simulink library "PES_CZ_FAW"  (Simulink 7.5)
settings: Solver=FixedStepDiscrete  StartTime=0.0  StopTime=10.0  FixedStep=0.01  MaxStep=0.01  RelTol=1e-3
undefined symbols (not defined in the file or in its folder): DiscIntNeverNeededParam, p_DRC_LoPsFilActPwr_s, p_DRC_LoPsFilPwrTi_s, p_DRC_LPFiltIC2_Tau_s, p_DRC_LPFiltIC2_Ts_s, p_DRC_LPFiltIC_Tau_s, p_DRC_LPFiltIC_Ts_s, Slope1, Slope2
libraries: BaseOperationLib_Browser x128, simulink x1
(part 1 of 2)
settings Model: Creator=ppr00086  LastModifiedBy=ppr00086

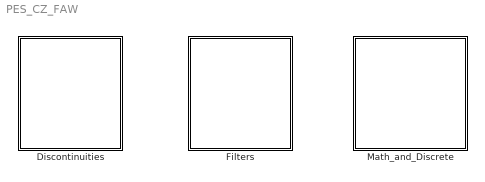
== system PES_CZ_FAW ==
  Discontinuities : Subsystem
  Filters : Subsystem  AncestorBlock=PES_CZ_FAW/Discontinuities
  Math_and_Discrete : Subsystem

== system PES_CZ_FAW/Discontinuities ==
  GetBit : Subsystem  mask{maska=16}
      mask prompts: maska "bitAND with parameter"
      mask help:
      | Get Bit
      |
      | Implements Masked AND between the input and mask. If the result is grater than zero true is set to output - otherwise false.
      |
      | Block is useful for decoding bit-encoded data.
      |
      | Mask may not be a calibratable parameter.
      mask Help:
      | Get Bit
      | 
      | Implements Masked AND between the input and mask. If the result is grater than zero true is set to output - otherwise false.
      | 
      | Block is useful for decoding bit-encoded data.
      | 
      | Mask may not be a calibratable parameter.
      mask Display: disp(['Input bitAND \n',maska]);
  Relay : Subsystem  mask{Thresshold=50, Hysteresis=5}
      mask help:
      | Block implements the relay functionality.
      |
      | Output is equal to one, when input is bigger or equal to Thresshold.
      | Output is equal to zero, when input is lower than (Thresshold - Hysteresis)
      | Otherwise, current output is equal to previous output.
      mask Help:
      | Block implements the relay functionality.
      | 
      | Output is equal to one, when input is bigger or equal to Thresshold.
      | Output is equal to zero, when input is lower than (Thresshold - Hysteresis)
      | Otherwise, current output is equal to previous output.
      mask Display: disp(['Relay']);
  SetBit : Subsystem  mask{maska=16}
      mask prompts: maska "Set to value"
      mask help:
      | Set Bit
      |
      | Sets the bit specified by value if the input is greater than zero.
      |
      | Block is useful for encoding bit-encoded data.
      |
      | "Set to value" may not be a calibratable parameter.
      mask Help:
      | Set Bit
      | 
      | Sets the bit specified by value if the input is greater than zero.
      | 
      | Block is useful for encoding bit-encoded data.
      | 
      | "Set to value" may not be a calibratable parameter.
      mask Display: disp(['SetBit \n',maska]);
  WrapToVal : Subsystem  mask{Max=1, Min=-1, Wrap=0}
      mask prompts: Wrap "WRAP TO VALUE"
      mask help: If the input is above the MAX or is less then MIN, the output is set to WRAP TO VALUE, otherwise the output equals the input.
      mask Display: disp('WrapTo', 'texmode', 'on');
  WtchDog : Subsystem  mask{timeoutthres=[]}
      mask prompts: timeoutthres "Timeout counter Treshold"
      mask help:
      | WatchDog block
      |
      | If input bool signal is false for the number of step bigger than "Timeout counter Threshold" the output WatchDog signal is set to True.
      |
      | Tip. Set the thresshold to the required time in seconds devided by algorithm sampling time.
      mask Help:
      | WatchDog block
      | 
      | If input bool signal is false for the number of step bigger than "Timeout counter Threshold" the output WatchDog signal is set to True.
      | 
      | Tip. Set the thresshold to required time in second devided by sampling time.
  valid_check : Subsystem  mask(Validity check      ){init=0}
      mask prompts: init "Init value"
      mask help:
      | Block checks, if the signal is valid. If not, signal is replaced by its
      | last valid value.
      mask Help:
      | Block checks, if the signal is valid. If not, signal is replaced by its
      | last valid value.

== system PES_CZ_FAW/Filters ==
  LPFilt : Subsystem  mask(Low-Pass filter){Ts=p_DRC_LoPsFilPwrTi_s, Tau=p_DRC_LoPsFilActPwr_s}
      mask prompts: Ts "Sampling Time Ts [s]"; Tau "Time constant Tau [s]"
      mask help:
      | Discrete low-pass filter of the first order that corresponds to continuous filter:
      |
      | T(s) = 1 / (Tau*s + 1)
      |
      | Filter is implemented using backward Euler discretization with sampling period Ts.
      |
      | For best results Tau and Ts should fullfill
      | Tau > 10 * Ts
      |
      | Note: Sampling rate of the filter inherrits the sampling rate of the input. This provides the compatibility with triggered subsystems.
      mask init:
      | if Ts*3>Tau,
      |    warndlg('Tau should be at least 3x higher than Ts')
      | end
      | 
      | if Tau<0,
      |    error('Tau must be greater than zero.')
      | end
      | 
      | if Ts<=0,
      |    error('Ts must be greater than zero.')
      | end
      settings: RTWSystemCode=Function  FunctionWithSeparateData=on
      mask Help:
      | Discrete low-pass filter of the first order that corresponds to continuous filter:
      | 
      | T(s) = 1 / (Tau*s + 1)
      | 
      | Filter is implemented using backward Euler discretization with sampling period Ts.
      | 
      | For best results Tau and Ts should fullfill
      | Tau > 10 * Ts
      | 
      | Note: Sampling rate of the filter inherrits the sampling rate of the input. This provides the compatibility with triggered subsystems.
      mask Display:
      | text(0.1,0.8,'1st order lowpass filter')
      | 
      | port_label('input',1,'u(t)')
      | 
      | port_label('output',1,'y(t)')
  LPFiltIC : Subsystem  mask(Low-Pass filter with external Initial Conditions){Ts=p_DRC_LPFiltIC_Ts_s, Tau=p_DRC_LPFiltIC_Tau_s}
      mask prompts: Ts "Sampling Time Ts [s]"; Tau "Time constant Tau [s]"
      mask help:
      | Discrete low-pass filter of the first order with external initial conditions that corresponds to continuous filter:
      |
      | T(s) = 1 / (Tau*s + 1)
      |
      | Filter is implemented using backward Euler discretization with sampling period Ts.
      |
      | For best results Tau and Ts should fullfill
      | Tau > 10 * Ts
      |
      | Note: Sampling rate of the filter inherrits the sampling rate of the input. This provides the compatibility with triggered subsystems.
      mask init:
      | if Ts*3>Tau,
      |    warndlg('Tau should be at least 3x higher than Ts')
      | end
      | 
      | if Tau<0,
      |    error('Tau must be greater than zero.')
      | end
      | 
      | if Ts<=0,
      |    error('Ts must be greater than zero.')
      | end
      settings: RTWSystemCode=Function  FunctionWithSeparateData=on
      mask Help:
      | Discrete low-pass filter of the first order that corresponds to continuous filter:
      | 
      | T(s) = 1 / (Tau*s + 1)
      | 
      | Filter is implemented using backward Euler discretization with sampling period Ts.
      | 
      | For best results Tau and Ts should fullfill
      | Tau > 10 * Ts
      | 
      | Note: Sampling rate of the filter inherrits the sampling rate of the input. This provides the compatibility with triggered subsystems.
      mask Display:
      | text(0.2,0.8,'1st order lowpass with IC');
      | 
      | port_label('input',1,'u(t)')
      | port_label('input',2,'IC')
      | port_label('output',1,'y(t)')
  LPFiltICEnRst : Subsystem  mask(Low-Pass filter Enabled Resettable External Initial Condition){Ts=p_DRC_LPFiltIC2_Ts_s, Tau=p_DRC_LPFiltIC2_Tau_s}
      mask prompts: Ts "Sampling Time Ts [s]"; Tau "Time constant Tau [s]"
      mask help:
      | Discrete low-pass filter of the first order with external initial conditions that corresponds to continuous filter:
      |
      | T(s) = 1 / (Tau*s + 1)
      |
      | Filter is implemented using backward Euler discretization with sampling period Ts.
      |
      | For best results Tau and Ts should fullfill
      | Tau > 10 * Ts
      |
      | The block is enabled, when the Enable input is equal to 1. The reset of the block is executed when the Reset input is set from 0 to 1.
      |
      | Note: Sampling rate of the filter inherrits the sampling rate of the input. This provides the compatibility with triggered subsystems.
      mask init:
      | if Ts*3>Tau,
      |    warndlg('Tau should be at least 3x higher than Ts')
      | end
      | 
      | if Tau<0,
      |    error('Tau must be greater than zero.')
      | end
      | 
      | if Ts<=0,
      |    error('Ts must be greater than zero.')
      | end
      mask Help:
      | Discrete low-pass filter of the first order that corresponds to continuous filter:
      | 
      | T(s) = 1 / (Tau*s + 1)
      | 
      | Filter is implemented using backward Euler discretization with sampling period Ts.
      | 
      | For best results Tau and Ts should fullfill
      | Tau > 10 * Ts
      | 
      | Note: Sampling rate of the filter inherrits the sampling rate of the input. This provides the compatibility with triggered subsystems.
      mask Display:
      | text(0.35,0.8,'1st order lowpass with IC');
      | text(0.35,0.25,strcat('Ts =',32,num2str(Ts),'s'));
      | text(0.35,0.5,strcat('Tau =',32,num2str(Tau),'s'));
      | 
      | port_label('input',1,'u(t)');
      | port_label('input',2,'IC')
      | port_label('output',1,'y(t)')
      | port_label('input',3,'Enable')
      | port_label('input',4,'Reset')
  LPFiltRst : Subsystem  mask(Low-Pass filter Resettable){Ts=[], Tau=[]}
      mask prompts: Ts "Sampling Time Ts [s]"; Tau "Time constant Tau [s]"
      mask help:
      | Discrete low-pass filter of the first order that corresponds to continuous filter:
      |
      | T(s) = 1 / (Tau*s + 1)
      |
      | Filter is implemented using backward Euler discretization with sampling period Ts.
      |
      | For best results Tau and Ts should fullfill
      | Tau > 10 * Ts
      |
      | Note: Sampling rate of the filter inherrits the sampling rate of the input. This provides the compatibility with triggered subsystems.
      mask init:
      | if Ts*3>Tau,
      |    warndlg('Tau should be at least 3x higher than Ts')
      | end
      | 
      | if Tau<0,
      |    error('Tau must be greater than zero.')
      | end
      | 
      | if Ts<=0,
      |    error('Ts must be greater than zero.')
      | end
      settings: RTWSystemCode=Function  FunctionWithSeparateData=on
      mask Help:
      | Discrete low-pass filter of the first order that corresponds to continuous filter:
      | 
      | T(s) = 1 / (Tau*s + 1)
      | 
      | Filter is implemented using backward Euler discretization with sampling period Ts.
      | 
      | For best results Tau and Ts should fullfill
      | Tau > 10 * Ts
      | 
      | Note: Sampling rate of the filter inherrits the sampling rate of the input. This provides the compatibility with triggered subsystems.
      mask Display:
      | text(0.25,0.8,'1st order lowpass');
      | text(0.25,0.25,strcat('Ts =',32,num2str(Ts),'s'));
      | text(0.25,0.5,strcat('Tau =',32,num2str(Tau),'s'));
  discrete_filter : Subsystem  mask(Discrete filter (first order)){num1=0, num2=0, den1=0, den2=0}
      mask prompts: num1 "num 1"; num2 "num 2"; den1 "den 1"; den2 "den 2"
      mask help:
      | num1*z + num2
      | Y(k) =  ------------------
      |            den1*z + den2
      mask Help:
      | num1*z + num2
      | Y(k) =  ------------------
      |            den1*z + den2
      mask Display:
      | port_label('input', 1, 'u(z)')
      | port_label('output', 1, 'y(z)')

== system PES_CZ_FAW/Math_and_Discrete ==
  Compare To Constant : Subsystem  mask(Compare To Constant){relop=<=, const=3.0, LogicOutDataTypeMode=uint8, ZeroCross=on}
      mask prompts: relop "Operator:"; const "Constant value:"; LogicOutDataTypeMode "Output data type mode:"; ZeroCross "Enable zero-crossing detection"
      mask help: Determine how a signal compares to a constant.
      mask init:
      | blkName = gcb;
      | 
      | if strcmp(get_param(gcbh,'LogicOutDataTypeMode'),'boolean')
      | 	setValue = 'Boolean';
      | else
      | 	setValue = 'Specify via dialog';
      | end
      | 
      | set_param([blkName,'/Compare'],'relop',relop, ...
      | 	'LogicOutDataTypeMode', setValue, 'ZeroCross', ZeroCross);
      | 
      | str = [relop,' C']; %default
      | 
      | const_str = get_param(blkName, 'const');
      | 
      | if isempty(strfind(const_str, ' ')) && isempty(strfind(const_str, ','))
      |     % scalar or single expression
      |     if isempty(str2num(const_str))
      |         %expression
      |         str = [relop, ' ', const_str];
      |     elseif length(const) == 1
      |         str = [relop,' ',num2str(double(const))];
      |     end
      | end
      mask StyleString: popup(==|~=|<|<=|>=|>),edit,popup(uint8|boolean),checkbox
      mask CallbackString: |||sl('zeroCrossEnable', gcbh);
      mask Display: disp(num2str(const));
  Compare To Zero : Subsystem  mask(Compare To Zero){relop=<=, LogicOutDataTypeMode=uint8, ZeroCross=on}
      mask prompts: relop "Operator:"; LogicOutDataTypeMode "Output data type mode:"; ZeroCross "Enable zero-crossing detection"
      mask help: Determine how a signal compares to zero.
      mask init:
      | blkName = gcb;
      | 
      | if strcmp(get_param(gcbh,'LogicOutDataTypeMode'),'boolean')
      | 	setValue = 'Boolean';
      | else
      |     setValue = 'Specify via dialog';
      | end
      | 
      | set_param([blkName,'/Compare'],'relop',relop, ...
      | 	'LogicOutDataTypeMode', setValue, 'ZeroCross', ZeroCross);
      mask StyleString: popup(==|~=|<|<=|>=|>),popup(uint8|boolean),checkbox
      mask CallbackString: ||sl('zeroCrossEnable', gcbh);
      mask Display: disp([relop,' 0'])
  Detect Decrease : Subsystem  mask(Detect Decrease){vinit=0.0}
      mask prompts: vinit "Initial condition:"
      mask help: If the input is strictly less than its previous value, then output TRUE, otherwise output FALSE. The initial condition determines the initial value of the previous input U/z.
      mask Display: fprintf('U < U/z')
  "Range Check " : Subsystem  mask(Range Checker){Min=0, Max=10}
      mask prompts: Min "Minumim"; Max "Maximum"
      mask help: Simple signal range check block. Checks whether the input signal falls into <Min,Max> interval.
      mask Help: Simple signal range check block. Checks whether the input signal falls into <Min,Max> interval.
  Rate Limiter Dynamic : Subsystem
      mask Type: Rate Limiter Dynamic
      mask Description: Limit rising and falling rates of the signals at the second input by using the first input (upper limit) and the third input (lower limit).
      mask Display: plot([0.15 0.95],[.5 .5],[.5 .5],[0.05 0.95],0.05+0.9*[.2 .8],0.05+0.9*[0 1]);
  Unit Delay Resettable : Subsystem  mask(Unit Delay Resettable){vinit=0, tsamp=-1}
      mask prompts: vinit "Initial Condition"; tsamp "Sample Time"
      mask help: Unit Delay Resettable
      mask Display: dpoly(1,[1 0],'z')

== system PES_CZ_FAW/Discontinuities/GetBit ==
  In1 : Inport  OutDataType=fixdt(1, 16)  OutScaling=2^0
  Bitwise Operator : S-Function  FunctionName=sfix_bitop  Parameters=UseBitMask,NumInputPorts,BitMask,BitMaskRealWorld,logicop  EnableBusSupport=off  mask(Bitwise Operator){logicop=AND, UseBitMask=on, NumInputPorts=1, BitMask=eval(maska), BitMaskRealWorld=Stored Integer}
      mask prompts: logicop "Operator:"; UseBitMask "Use bit mask ..."; NumInputPorts "Number of input ports:"; BitMask "Bit Mask"; BitMaskRealWorld "Treat mask as:"
      mask help: Perform the specified bitwise operation on the inputs. The output data type should represent zero exactly.
      mask init:
      | str = '';
      | if UseBitMask
      |   [m,n] = size(BitMask);
      |   if ischar(BitMask)
      |     len = m;
      |     n = 1;
      |   else
      |     len = m * n;
      |   end
      |   internalBitMask = zeros(m,n);
      |   if isnumeric(BitMask)
      |     for i=1:len,
      |       internalBitMask(i) = BitMask(i);
      |     end
      |   elseif ischar(BitMask)
      |     for i=1:m,
      |       internalBitMask(i) = hex2dec(BitMask(i,:));
      |     end
      |   elseif iscell(BitMask)
      |     for i=1:len,
      |       if isnumeric( BitMask{i} )
      |         internalBitMask(i) = BitMask{i};
      |       elseif ischar( BitMask{i} )
      |         internalBitMask(i) = hex2dec(BitMask{i});
      |       else
      |         errordlg(['Data type is not supported at cell item ', num2str(i) ]);
      |       end
      |     end
      |   end
      |   BitMask = internalBitMask;
      |   for i=1:len
      |     if BitMask(i) > (2^52)-1
      |       error(DAStudio.message('Simulink:blocks:BitMaskWordLengthTooLarge')); 
      |     end
      |   end 
      |   if len == 1
      |      if BitMaskRealWorld == 1 || BitMask(1) < 0
      |        str=num2str(BitMask(1));
      |      else
      |        str=['0x',dec2hex(floor(BitMask(1)))];
      |      end
      |   else
      |      str='Masks';
      |   end
      | else
      |   BitMask = 0;
      |   str='';
      | end
      mask StyleString: popup(AND|OR|NAND|NOR|XOR|NOT),checkbox,edit,edit,popup(Real World Value|Stored Integer)
      mask CallbackString: fixptdialog(gcbh)|fixptdialog(gcbh)|||
      mask Display: fprintf(['Bitwise\n',logicop,'\n',str])
  Compare To Constant : BaseOperationLib_Browser/Logic Operations Changed/Compare To Constant  SystemSampleTime=-1  relop=>  const=0
  Out1 : Outport  OutDataType=fixdt(1, 16)  OutScaling=2^0
  wires:
  In1/1 -> Bitwise Operator/1
  Bitwise Operator/1 -> Compare To Constant/1
  Compare To Constant/1 -> Out1/1

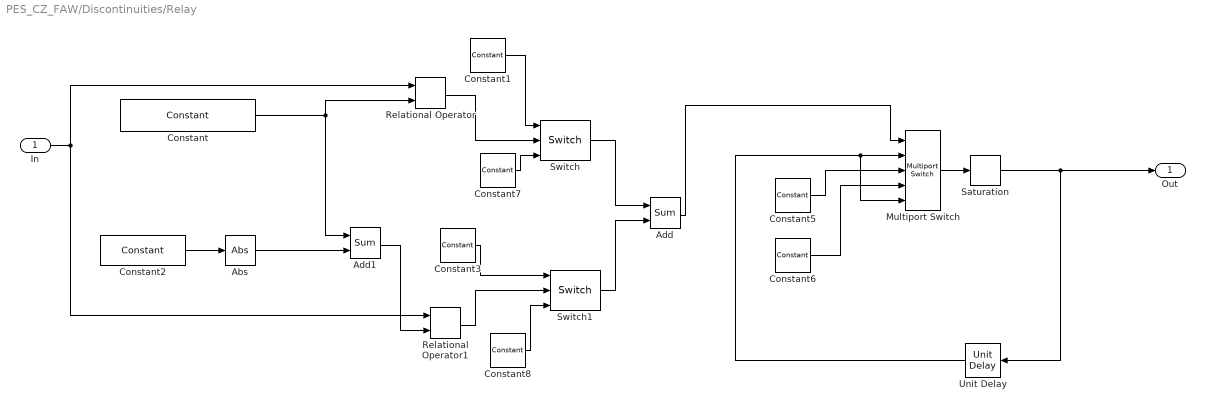
== system PES_CZ_FAW/Discontinuities/Relay ==
  In : Inport
  Abs : BaseOperationLib_Browser/Math Operations Changed/Abs  OutMax=[]  OutDataType=fixdt(1, 16)  OutScaling=2^0
  Add : BaseOperationLib_Browser/Math Operations Changed/Sum  Inputs=++  OutMin=[]  OutMax=[]  OutDataType=fixdt(1, 16)  OutScaling=2^0
  Add1 : BaseOperationLib_Browser/Math Operations Changed/Sum  Inputs=+-  OutMin=[]  OutMax=[]  OutDataType=fixdt(1, 16)  OutScaling=2^0
  Constant : BaseOperationLib_Browser/Sources&Sinks/Constant  Value=Thresshold  OutMin=[]  OutMax=[]  OutDataType=fixdt(1, 16)  ConRadixGroup=Use specified scaling  OutScaling=2^0  OutDataTypeStr=Inherit: Inherit from 'Constant value'
  Constant1 : BaseOperationLib_Browser/Sources&Sinks/Constant  Value=1  OutMin=[]  OutMax=[]  OutDataType=fixdt(1, 16)  ConRadixGroup=Use specified scaling  OutScaling=2^0  OutDataTypeStr=Inherit: Inherit from 'Constant value'
  Constant2 : BaseOperationLib_Browser/Sources&Sinks/Constant  Value=Hysteresis  OutMin=[]  OutMax=[]  OutDataType=fixdt(1, 16)  ConRadixGroup=Use specified scaling  OutScaling=2^0  OutDataTypeStr=Inherit: Inherit from 'Constant value'
  Constant3 : BaseOperationLib_Browser/Sources&Sinks/Constant  Value=2  OutMin=[]  OutMax=[]  OutDataType=fixdt(1, 16)  ConRadixGroup=Use specified scaling  OutScaling=2^0  OutDataTypeStr=Inherit: Inherit from 'Constant value'
  Constant5 : BaseOperationLib_Browser/Sources&Sinks/Constant  Value=1  OutMin=[]  OutMax=[]  OutDataType=fixdt(1, 16)  ConRadixGroup=Use specified scaling  OutScaling=2^0  OutDataTypeStr=Inherit: Inherit from 'Constant value'
  Constant6 : BaseOperationLib_Browser/Sources&Sinks/Constant  Value=0  OutMin=[]  OutMax=[]  OutDataType=fixdt(1, 16)  ConRadixGroup=Use specified scaling  OutScaling=2^0  OutDataTypeStr=Inherit: Inherit from 'Constant value'
  Constant7 : BaseOperationLib_Browser/Sources&Sinks/Constant  Value=0  OutMin=[]  OutMax=[]  OutDataType=fixdt(1, 16)  ConRadixGroup=Use specified scaling  OutScaling=2^0  OutDataTypeStr=Inherit: Inherit from 'Constant value'
  Constant8 : BaseOperationLib_Browser/Sources&Sinks/Constant  Value=0  OutMin=[]  OutMax=[]  OutDataType=fixdt(1, 16)  ConRadixGroup=Use specified scaling  OutScaling=2^0  OutDataTypeStr=Inherit: Inherit from 'Constant value'
  Multiport Switch : BaseOperationLib_Browser/Signal Routing Changed/Multiport Switch  DataPortOrder=Zero-based contiguous  Inputs=4  DataPortIndices={1,2,3}  zeroidx=on  OutMin=[]  OutMax=[]  OutDataType=fixdt(1, 16)  OutScaling=2^0
  Relational Operator : BaseOperationLib_Browser/Logic Operations Changed/Relational Operator  Operator=>=  LogicOutDataTypeMode=boolean  LogicDataType=PDT_Bool  OutDataTypeStr=boolean
  Relational Operator1 : BaseOperationLib_Browser/Logic Operations Changed/Relational Operator  Operator=<  LogicOutDataTypeMode=boolean  LogicDataType=PDT_Bool  OutDataTypeStr=boolean
  Saturation : BaseOperationLib_Browser/Discontinuities Unchanged/Saturation  UpperLimit=1  LowerLimit=0  OutMin=[]  OutMax=[]  OutDataType=fixdt(1, 16)  OutScaling=2^0
      settings: AttributesFormatString=ULim:%<UpperLimit>\nLLim:%<LowerLimit>
  Switch : BaseOperationLib_Browser/Signal Routing Changed/Switch  Criteria=u2 ~= 0  Threshold=0  OutMin=[]  OutMax=[]  OutDataType=fixdt(1,16,0)  OutScaling=[]
  Switch1 : BaseOperationLib_Browser/Signal Routing Changed/Switch  Criteria=u2 ~= 0  Threshold=0  OutMin=[]  OutMax=[]  OutDataType=fixdt(1,16,0)  OutScaling=[]
  Unit Delay : BaseOperationLib_Browser/Discrete Unchanged /Unit Delay  X0=0  SampleTime=-1
  Out : Outport
  wires:
  In/1 -> Relational Operator/1, Relational Operator1/1
  Constant/1 -> Add1/1, Relational Operator/2
  Relational Operator/1 -> Switch/2
  Constant1/1 -> Switch/1
  Relational Operator1/1 -> Switch1/2
  Constant3/1 -> Switch1/1
  Switch/1 -> Add/1
  Switch1/1 -> Add/2
  Add/1 -> Multiport Switch/1
  Abs/1 -> Add1/2
  Constant2/1 -> Abs/1
  Constant5/1 -> Multiport Switch/3
  Multiport Switch/1 -> Saturation/1
  Constant6/1 -> Multiport Switch/4
  Constant7/1 -> Switch/3
  Constant8/1 -> Switch1/3
  Unit Delay/1 -> Multiport Switch/2, Multiport Switch/5
  Saturation/1 -> Unit Delay/1, Out/1
  Add1/1 -> Relational Operator1/2

== system PES_CZ_FAW/Discontinuities/SetBit ==
  In1 : Inport  OutDataType=fixdt(1, 16)  OutScaling=2^0
  Compare To Constant : BaseOperationLib_Browser/Logic Operations Changed/Compare To Constant  SystemSampleTime=-1  relop=>  const=0
  Data Type Conversion : DataTypeConversion  OutDataTypeMode=uint32  OutDataType=fixdt(1, 16)  OutScaling=2^0  OutDataTypeStr=uint32
  Gain : BaseOperationLib_Browser/Math Operations Changed/Gain  Gain=uint32(eval(maska))  Multiplication=Element-wise(K.*u)  ParamMin=[]  ParamMax=[]  ParameterDataType=fixdt(1, 16)  ParameterScalingMode=Best Precision: Matrix-wise  ParameterScaling=2^0  ParamDataTypeStr=Inherit: Inherit from 'Gain'  OutMin=[]  OutMax=[]  OutDataType=fixdt(1, 16)  OutScaling=2^0  SaturateOnIntegerOverflow=on
  Out1 : Outport  OutDataType=fixdt(1, 16)  OutScaling=2^0
  wires:
  Compare To Constant/1 -> Data Type Conversion/1
  Gain/1 -> Out1/1
  In1/1 -> Compare To Constant/1
  Data Type Conversion/1 -> Gain/1

== system PES_CZ_FAW/Discontinuities/WrapToVal ==
  In1 : Inport  OutDataType=fixdt(1, 16)  OutScaling=2^0
  Compare To Constant : BaseOperationLib_Browser/Logic Operations Changed/Compare To Constant  SystemSampleTime=-1  relop=<=  const=Max
  Compare To Constant1 : BaseOperationLib_Browser/Logic Operations Changed/Compare To Constant  SystemSampleTime=-1  relop=>=  const=Min
  Constant : BaseOperationLib_Browser/Sources&Sinks/Constant  Value=Wrap  OutMin=[]  OutMax=[]  OutDataType=fixdt(1, 16)  ConRadixGroup=Use specified scaling  OutScaling=2^0  OutDataTypeStr=Inherit: Inherit via back propagation
  Logical Operator : BaseOperationLib_Browser/Logic Operations Changed/Logical Operator  Operator=AND  Inputs=2  AllPortsSameDT=on  OutDataTypeMode=Specify via dialog  LogicDataType=PDT_Bool  OutDataTypeStr=PDT_Bool
  Switch : BaseOperationLib_Browser/Signal Routing Changed/Switch  Criteria=u2 ~= 0  Threshold=1  InputSameDT=on  OutMin=[]  OutMax=[]  OutDataType=fixdt(1,16,0)  OutScaling=[]  SaturateOnIntegerOverflow=on
  Out1 : Outport  OutDataType=fixdt(1, 16)  OutScaling=2^0
  wires:
  In1/1 -> Compare To Constant1/1, Compare To Constant/1, Switch/1
  Switch/1 -> Out1/1
  Constant/1 -> Switch/3
  Logical Operator/1 -> Switch/2
  Compare To Constant1/1 -> Logical Operator/2
  Compare To Constant/1 -> Logical Operator/1

== system PES_CZ_FAW/Discontinuities/WtchDog ==
  ValidSig : Inport  OutDataType=fixdt(1, 16)  OutScaling=2^0
  Constant : BaseOperationLib_Browser/Sources&Sinks/Constant  Value=timeoutthres  OutMin=[]  OutMax=[]  OutDataType=fixdt(1, 16)  ConRadixGroup=Use specified scaling  OutScaling=2^0  OutDataTypeStr=Inherit: Inherit from 'Constant value'
  Discrete-Time Integrator1 : DiscreteIntegrator  IntegratorMethod=Integration: Backward Euler  ExternalReset=rising  SampleTime=-1  OutDataType=PDT_s  OutDataTypeStr=Inherit: Inherit via back propagation  UpperSaturationLimit=100  LowerSaturationLimit=0  ICPrevOutput=DiscIntNeverNeededParam  ICPrevScaledInput=DiscIntNeverNeededParam
  Logical Operator : BaseOperationLib_Browser/Logic Operations Changed/Logical Operator  Operator=AND  Inputs=2  AllPortsSameDT=on  OutDataTypeMode=Specify via dialog  LogicDataType=PDT_Bool  OutDataTypeStr=PDT_Bool
  Logical Operator2 : BaseOperationLib_Browser/Logic Operations Changed/Logical Operator  Operator=NOT  Inputs=2  AllPortsSameDT=on  OutDataTypeMode=Specify via dialog  LogicDataType=PDT_Bool  OutDataTypeStr=PDT_Bool
  Relational Operator : BaseOperationLib_Browser/Logic Operations Changed/Relational Operator  Operator=>=  InputSameDT=on  LogicOutDataTypeMode=Specify via dialog  LogicDataType=PDT_Bool  OutDataTypeStr=PDT_Bool
  WatchDogErr : Outport  OutDataType=fixdt(1, 16)  OutScaling=2^0
  wires:
  ValidSig/1 -> Logical Operator2/1
  Relational Operator/1 -> Logical Operator/1
  Logical Operator/1 -> WatchDogErr/1
  Constant/1 -> Relational Operator/2
  Discrete-Time Integrator1/1 -> Relational Operator/1
  Logical Operator2/1 -> Discrete-Time Integrator1/1, Discrete-Time Integrator1/2, Logical Operator/2

== system PES_CZ_FAW/Discontinuities/valid_check ==
  Signal : Inport
  Valid : Inport  Port=2
  Switch : BaseOperationLib_Browser/Signal Routing Changed/Switch  Criteria=u2 ~= 0  Threshold=1  InputSameDT=on  OutMin=[]  OutMax=[]  OutDataType=fixdt(1,16,0)  OutScaling=[]  SaturateOnIntegerOverflow=on
  Unit Delay : BaseOperationLib_Browser/Discrete Unchanged /Unit Delay  X0=init  SampleTime=-1
  SignalOut : Outport
  wires:
  Switch/1 -> Unit Delay/1, SignalOut/1
  Unit Delay/1 -> Switch/3
  Signal/1 -> Switch/1
  Valid/1 -> Switch/2

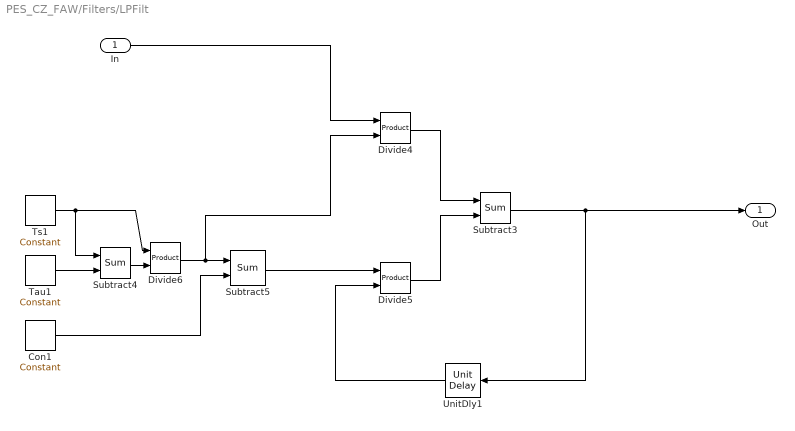
== system PES_CZ_FAW/Filters/LPFilt ==
  In : Inport
  Con1 : BaseOperationLib_Browser/Sources&Sinks/Constant  Value=1  OutMin=[]  OutMax=[]  OutDataType=fixdt(1, 16)  ConRadixGroup=Use specified scaling  OutScaling=2^0  OutDataTypeStr=Inherit: Inherit from 'Constant value'
  Divide4 : BaseOperationLib_Browser/Math Operations Changed/Product  Inputs=**  Multiplication=Element-wise(.*)  OutMin=[]  OutMax=[]  OutDataType=fixdt(1,16,0)  OutScaling=[]
  Divide5 : BaseOperationLib_Browser/Math Operations Changed/Product  Inputs=**  Multiplication=Element-wise(.*)  OutMin=[]  OutMax=[]  OutDataType=fixdt(1,16,0)  OutScaling=[]
  Divide6 : BaseOperationLib_Browser/Math Operations Changed/Product  Inputs=*/  Multiplication=Element-wise(.*)  OutMin=[]  OutMax=[]  OutDataType=fixdt(1,16,0)  OutScaling=[]
  Subtract3 : BaseOperationLib_Browser/Math Operations Changed/Sum  Inputs=++  OutMin=[]  OutMax=[]  OutDataType=fixdt(1, 16)  OutScaling=2^0
  Subtract4 : BaseOperationLib_Browser/Math Operations Changed/Sum  Inputs=++  OutMin=[]  OutMax=[]  OutDataType=fixdt(1, 16)  OutScaling=2^0
  Subtract5 : BaseOperationLib_Browser/Math Operations Changed/Sum  Inputs=-+  OutMin=[]  OutMax=[]  OutDataType=fixdt(1, 16)  OutScaling=2^0
  Tau1 : BaseOperationLib_Browser/Sources&Sinks/Constant  Value=Tau  OutMin=[]  OutMax=[]  OutDataType=fixdt(1, 16)  ConRadixGroup=Use specified scaling  OutScaling=2^0  OutDataTypeStr=Inherit: Inherit from 'Constant value'
  Ts1 : BaseOperationLib_Browser/Sources&Sinks/Constant  Value=Ts  OutMin=[]  OutMax=[]  OutDataType=fixdt(1, 16)  ConRadixGroup=Use specified scaling  OutScaling=2^0  OutDataTypeStr=Inherit: Inherit from 'Constant value'
  UnitDly1 : BaseOperationLib_Browser/Discrete Unchanged /Unit Delay  X0=0  SampleTime=-1
  Out : Outport
  wires:
  Subtract5/1 -> Divide5/1
  Tau1/1 -> Subtract4/2
  Ts1/1 -> Subtract4/1, Divide6/1
  Subtract4/1 -> Divide6/2
  Divide6/1 -> Divide4/2, Subtract5/1
  Con1/1 -> Subtract5/2
  In/1 -> Divide4/1
  Divide4/1 -> Subtract3/1
  UnitDly1/1 -> Divide5/2
  Divide5/1 -> Subtract3/2
  Subtract3/1 -> Out/1, UnitDly1/1

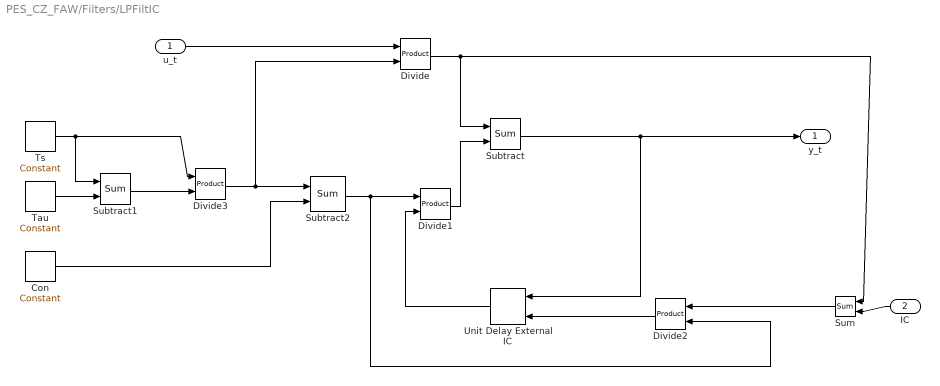
== system PES_CZ_FAW/Filters/LPFiltIC ==
  u_t : Inport
  IC : Inport  Port=2
  Con : BaseOperationLib_Browser/Sources&Sinks/Constant  Value=1  OutMin=[]  OutMax=[]  OutDataType=fixdt(1, 16)  ConRadixGroup=Use specified scaling  OutScaling=2^0  OutDataTypeStr=Inherit: Inherit from 'Constant value'
  Divide : BaseOperationLib_Browser/Math Operations Changed/Product  Inputs=**  Multiplication=Element-wise(.*)  OutMin=[]  OutMax=[]  OutDataType=fixdt(1,16,0)  OutScaling=[]
  Divide1 : BaseOperationLib_Browser/Math Operations Changed/Product  Inputs=**  Multiplication=Element-wise(.*)  OutMin=[]  OutMax=[]  OutDataType=fixdt(1,16,0)  OutScaling=[]
  Divide2 : BaseOperationLib_Browser/Math Operations Changed/Product  Inputs=*/  Multiplication=Element-wise(.*)  OutMin=[]  OutMax=[]  OutDataType=fixdt(1,16,0)  OutScaling=[]
  Divide3 : BaseOperationLib_Browser/Math Operations Changed/Product  Inputs=*/  Multiplication=Element-wise(.*)  OutMin=[]  OutMax=[]  OutDataType=fixdt(1,16,0)  OutScaling=[]
  Subtract : BaseOperationLib_Browser/Math Operations Changed/Sum  Inputs=++  OutMin=[]  OutMax=[]  OutDataType=fixdt(1, 16)  OutScaling=2^0
  Subtract1 : BaseOperationLib_Browser/Math Operations Changed/Sum  Inputs=++  OutMin=[]  OutMax=[]  OutDataType=fixdt(1, 16)  OutScaling=2^0
  Subtract2 : BaseOperationLib_Browser/Math Operations Changed/Sum  Inputs=-+  OutMin=[]  OutMax=[]  OutDataType=fixdt(1, 16)  OutScaling=2^0
  Sum : BaseOperationLib_Browser/Math Operations Changed/Sum  Inputs=-+|  OutMin=[]  OutMax=[]  OutDataType=fixdt(1, 16)  OutScaling=2^0
  Tau : BaseOperationLib_Browser/Sources&Sinks/Constant  Value=Tau  OutMin=[]  OutMax=[]  OutDataType=fixdt(1, 16)  ConRadixGroup=Use specified scaling  OutScaling=2^0  OutDataTypeStr=Inherit: Inherit from 'Constant value'
  Ts : BaseOperationLib_Browser/Sources&Sinks/Constant  Value=Ts  OutMin=[]  OutMax=[]  OutDataType=fixdt(1, 16)  ConRadixGroup=Use specified scaling  OutScaling=2^0  OutDataTypeStr=Inherit: Inherit from 'Constant value'
  Unit Delay External IC : BaseOperationLib_Browser/Discrete Unchanged /Unit Delay External IC  SystemSampleTime=-1  tsamp=-1
  y_t : Outport
  wires:
  Tau/1 -> Subtract1/2
  Ts/1 -> Subtract1/1, Divide3/1
  Subtract1/1 -> Divide3/2
  Divide3/1 -> Divide/2, Subtract2/1
  Con/1 -> Subtract2/2
  Subtract2/1 -> Divide2/2, Divide1/1
  IC/1 -> Sum/2
  Sum/1 -> Divide2/1
  Divide2/1 -> Unit Delay External IC/2
  u_t/1 -> Divide/1
  Divide/1 -> Sum/1, Subtract/1
  Unit Delay External IC/1 -> Divide1/2
  Divide1/1 -> Subtract/2
  Subtract/1 -> Unit Delay External IC/1, y_t/1

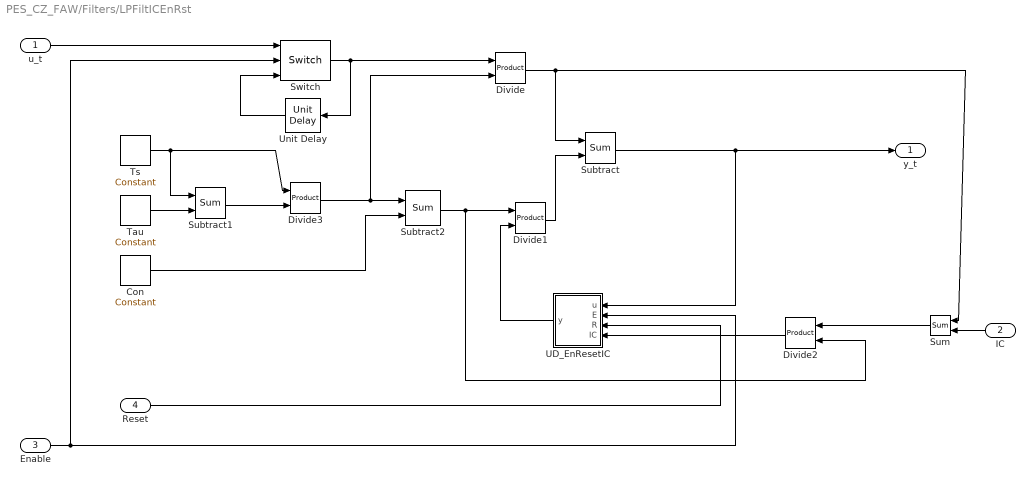
== system PES_CZ_FAW/Filters/LPFiltICEnRst ==
  u_t : Inport
  IC : Inport  Port=2
  Enable : Inport  Port=3
  Reset : Inport  Port=4
  Con : BaseOperationLib_Browser/Sources&Sinks/Constant  Value=1  OutMin=[]  OutMax=[]  OutDataType=fixdt(1, 16)  ConRadixGroup=Use specified scaling  OutScaling=2^0  OutDataTypeStr=Inherit: Inherit from 'Constant value'
  Divide : BaseOperationLib_Browser/Math Operations Changed/Product  Inputs=**  Multiplication=Element-wise(.*)  OutMin=[]  OutMax=[]  OutDataType=fixdt(1,16,0)  OutScaling=[]
  Divide1 : BaseOperationLib_Browser/Math Operations Changed/Product  Inputs=**  Multiplication=Element-wise(.*)  OutMin=[]  OutMax=[]  OutDataType=fixdt(1,16,0)  OutScaling=[]
  Divide2 : BaseOperationLib_Browser/Math Operations Changed/Product  Inputs=*/  Multiplication=Element-wise(.*)  OutMin=[]  OutMax=[]  OutDataType=fixdt(1,16,0)  OutScaling=[]
  Divide3 : BaseOperationLib_Browser/Math Operations Changed/Product  Inputs=*/  Multiplication=Element-wise(.*)  OutMin=[]  OutMax=[]  OutDataType=fixdt(1,16,0)  OutScaling=[]
  Subtract : BaseOperationLib_Browser/Math Operations Changed/Sum  Inputs=++  OutMin=[]  OutMax=[]  OutDataType=fixdt(1, 16)  OutScaling=2^0
  Subtract1 : BaseOperationLib_Browser/Math Operations Changed/Sum  Inputs=++  OutMin=[]  OutMax=[]  OutDataType=fixdt(1, 16)  OutScaling=2^0
  Subtract2 : BaseOperationLib_Browser/Math Operations Changed/Sum  Inputs=-+  OutMin=[]  OutMax=[]  OutDataType=fixdt(1, 16)  OutScaling=2^0
  Sum : BaseOperationLib_Browser/Math Operations Changed/Sum  Inputs=-+  OutMin=[]  OutMax=[]  OutDataType=fixdt(1, 16)  OutScaling=2^0
  Switch : BaseOperationLib_Browser/Signal Routing Changed/Switch  Criteria=u2 > Threshold  Threshold=0  OutMin=[]  OutMax=[]  OutDataType=fixdt(1,16,0)  OutScaling=[]
  Tau : BaseOperationLib_Browser/Sources&Sinks/Constant  Value=Tau  OutMin=[]  OutMax=[]  OutDataType=fixdt(1, 16)  ConRadixGroup=Use specified scaling  OutScaling=2^0  OutDataTypeStr=Inherit: Inherit from 'Constant value'
  Ts : BaseOperationLib_Browser/Sources&Sinks/Constant  Value=Ts  OutMin=[]  OutMax=[]  OutDataType=fixdt(1, 16)  ConRadixGroup=Use specified scaling  OutScaling=2^0  OutDataTypeStr=Inherit: Inherit from 'Constant value'
  UD_EnResetIC : Subsystem
  Unit Delay : BaseOperationLib_Browser/Discrete Unchanged /Unit Delay  X0=0  SampleTime=-1
  y_t : Outport
  wires:
  Con/1 -> Subtract2/2
  Divide3/1 -> Subtract2/1, Divide/2
  Subtract1/1 -> Divide3/2
  Ts/1 -> Divide3/1, Subtract1/1
  Tau/1 -> Subtract1/2
  Reset/1 -> UD_EnResetIC/3(R)
  Enable/1 -> Switch/2, UD_EnResetIC/2(E)
  Divide2/1 -> UD_EnResetIC/4(IC)
  Subtract/1 -> UD_EnResetIC/1(u), y_t/1
  Divide1/1 -> Subtract/2
  UD_EnResetIC/1(y) -> Divide1/2
  Divide/1 -> Subtract/1, Sum/1
  Sum/1 -> Divide2/1
  IC/1 -> Sum/2
  Subtract2/1 -> Divide1/1, Divide2/2
  Unit Delay/1 -> Switch/3
  u_t/1 -> Switch/1
  Switch/1 -> Divide/1, Unit Delay/1

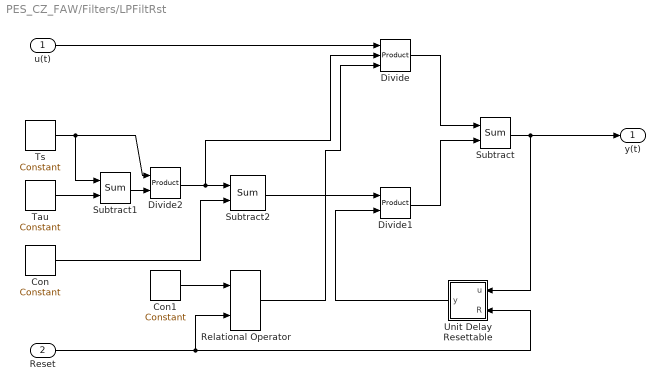
== system PES_CZ_FAW/Filters/LPFiltRst ==
  u(t) : Inport
  Reset : Inport  Port=2
  Con : BaseOperationLib_Browser/Sources&Sinks/Constant  Value=1  OutMin=[]  OutMax=[]  OutDataType=fixdt(1, 16)  ConRadixGroup=Use specified scaling  OutScaling=2^0  OutDataTypeStr=Inherit: Inherit from 'Constant value'
  Con1 : BaseOperationLib_Browser/Sources&Sinks/Constant  Value=0  OutMin=[]  OutMax=[]  OutDataType=fixdt(1, 16)  ConRadixGroup=Use specified scaling  OutScaling=2^0  OutDataTypeStr=Inherit: Inherit via back propagation
  Divide : BaseOperationLib_Browser/Math Operations Changed/Product  Inputs=***  Multiplication=Element-wise(.*)  OutMin=[]  OutMax=[]  OutDataType=fixdt(1,16,0)  OutScaling=[]
  Divide1 : BaseOperationLib_Browser/Math Operations Changed/Product  Inputs=**  Multiplication=Element-wise(.*)  OutMin=[]  OutMax=[]  OutDataType=fixdt(1,16,0)  OutScaling=[]
  Divide2 : BaseOperationLib_Browser/Math Operations Changed/Product  Inputs=*/  Multiplication=Element-wise(.*)  OutMin=[]  OutMax=[]  OutDataType=fixdt(1,16,0)  OutScaling=[]
  Relational Operator : BaseOperationLib_Browser/Logic Operations Changed/Relational Operator  Operator===  InputSameDT=on  LogicOutDataTypeMode=Specify via dialog  LogicDataType=PDT_Bool  OutDataTypeStr=PDT_Bool
  Subtract : BaseOperationLib_Browser/Math Operations Changed/Sum  Inputs=++  OutMin=[]  OutMax=[]  OutDataType=fixdt(1, 16)  OutScaling=2^0
  Subtract1 : BaseOperationLib_Browser/Math Operations Changed/Sum  Inputs=++  OutMin=[]  OutMax=[]  OutDataType=fixdt(1, 16)  OutScaling=2^0
  Subtract2 : BaseOperationLib_Browser/Math Operations Changed/Sum  Inputs=-+  OutMin=[]  OutMax=[]  OutDataType=fixdt(1, 16)  OutScaling=2^0
  Tau : BaseOperationLib_Browser/Sources&Sinks/Constant  Value=Tau  OutMin=[]  OutMax=[]  OutDataType=fixdt(1, 16)  ConRadixGroup=Use specified scaling  OutScaling=2^0  OutDataTypeStr=Inherit: Inherit from 'Constant value'
  Ts : BaseOperationLib_Browser/Sources&Sinks/Constant  Value=Ts  OutMin=[]  OutMax=[]  OutDataType=fixdt(1, 16)  ConRadixGroup=Use specified scaling  OutScaling=2^0  OutDataTypeStr=Inherit: Inherit from 'Constant value'
  Unit Delay Resettable : Subsystem
  y(t) : Outport
  wires:
  Con1/1 -> Relational Operator/1
  Relational Operator/1 -> Divide/3
  Subtract2/1 -> Divide1/1
  Tau/1 -> Subtract1/2
  Ts/1 -> Subtract1/1, Divide2/1
  Subtract1/1 -> Divide2/2
  Divide2/1 -> Divide/2, Subtract2/1
  Con/1 -> Subtract2/2
  u(t)/1 -> Divide/1
  Divide/1 -> Subtract/1
  Unit Delay Resettable/1(y) -> Divide1/2
  Divide1/1 -> Subtract/2
  Subtract/1 -> y(t)/1, Unit Delay Resettable/1(u)
  Reset/1 -> Relational Operator/2, Unit Delay Resettable/2(R)

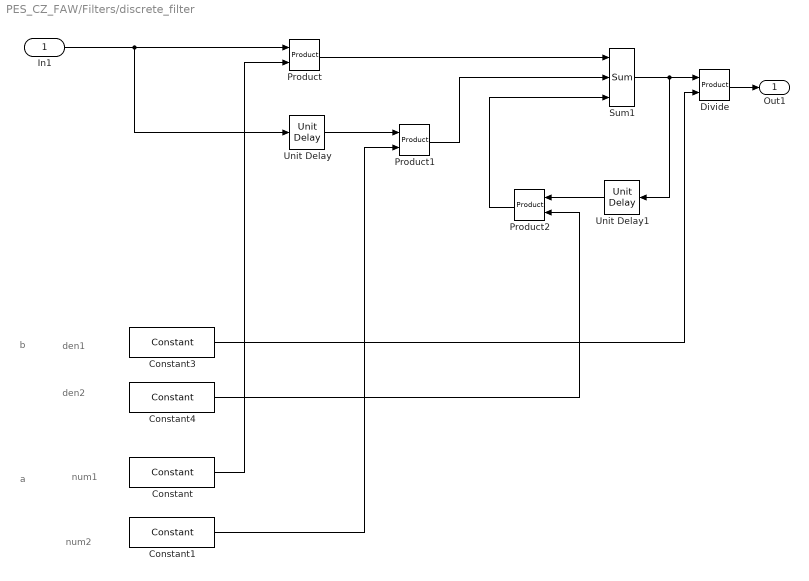
== system PES_CZ_FAW/Filters/discrete_filter ==
  note: b
  note: a
  note: den1
  note: den2
  note: num1
  note: num2
  In1 : Inport
  Constant : BaseOperationLib_Browser/Sources&Sinks/Constant  Value=num1  OutMin=[]  OutMax=[]  OutDataType=fixdt(1, 16)  ConRadixGroup=Use specified scaling  OutScaling=2^0  OutDataTypeStr=Inherit: Inherit from 'Constant value'
  Constant1 : BaseOperationLib_Browser/Sources&Sinks/Constant  Value=num2  OutMin=[]  OutMax=[]  OutDataType=fixdt(1, 16)  ConRadixGroup=Use specified scaling  OutScaling=2^0  OutDataTypeStr=Inherit: Inherit from 'Constant value'
  Constant3 : BaseOperationLib_Browser/Sources&Sinks/Constant  Value=den1  OutMin=[]  OutMax=[]  OutDataType=fixdt(1, 16)  ConRadixGroup=Use specified scaling  OutScaling=2^0  OutDataTypeStr=Inherit: Inherit from 'Constant value'
  Constant4 : BaseOperationLib_Browser/Sources&Sinks/Constant  Value=den2  OutMin=[]  OutMax=[]  OutDataType=fixdt(1, 16)  ConRadixGroup=Use specified scaling  OutScaling=2^0  OutDataTypeStr=Inherit: Inherit from 'Constant value'
  Divide : BaseOperationLib_Browser/Math Operations Changed/Product  Inputs=*/  Multiplication=Element-wise(.*)  OutMin=[]  OutMax=[]  OutDataType=fixdt(1,16,0)  OutScaling=[]
  Product : BaseOperationLib_Browser/Math Operations Changed/Product  Inputs=2  Multiplication=Element-wise(.*)  OutMin=[]  OutMax=[]  OutDataType=fixdt(1,16,0)  OutScaling=[]  OutDataTypeStr=Inherit: Inherit via back propagation  RndMeth=Zero  SaturateOnIntegerOverflow=on
  Product1 : BaseOperationLib_Browser/Math Operations Changed/Product  Inputs=2  Multiplication=Element-wise(.*)  OutMin=[]  OutMax=[]  OutDataType=fixdt(1,16,0)  OutScaling=[]  OutDataTypeStr=Inherit: Inherit via back propagation  RndMeth=Zero  SaturateOnIntegerOverflow=on
  Product2 : BaseOperationLib_Browser/Math Operations Changed/Product  Inputs=2  Multiplication=Element-wise(.*)  OutMin=[]  OutMax=[]  OutDataType=fixdt(1,16,0)  OutScaling=[]  OutDataTypeStr=Inherit: Inherit via back propagation  RndMeth=Zero  SaturateOnIntegerOverflow=on
  Sum1 : BaseOperationLib_Browser/Math Operations Changed/Sum  Inputs=++-  InputSameDT=on  OutMin=[]  OutMax=[]  OutDataType=fixdt(1, 16)  OutScaling=2^0  SaturateOnIntegerOverflow=on
  Unit Delay : BaseOperationLib_Browser/Discrete Unchanged /Unit Delay  X0=0  SampleTime=-1
  Unit Delay1 : BaseOperationLib_Browser/Discrete Unchanged /Unit Delay  X0=0  SampleTime=-1
  Out1 : Outport
  wires:
  Divide/1 -> Out1/1
  Constant3/1 -> Divide/2
  Product2/1 -> Sum1/3
  Constant4/1 -> Product2/2
  Unit Delay1/1 -> Product2/1
  Sum1/1 -> Divide/1, Unit Delay1/1
  Product1/1 -> Sum1/2
  Product/1 -> Sum1/1
  Constant1/1 -> Product1/2
  Unit Delay/1 -> Product1/1
  Constant/1 -> Product/2
  In1/1 -> Unit Delay/1, Product/1

== system PES_CZ_FAW/Math_and_Discrete/Compare To Constant ==
  u : Inport
  Constant : BaseOperationLib_Browser/Sources&Sinks/Constant  Value=const  OutMin=[]  OutMax=[]  OutDataType=fixdt(1, 16)  ConRadixGroup=Use specified scaling  OutScaling=2^0  OutDataTypeStr=Inherit: Inherit from 'Constant value'
  Relational Operator : BaseOperationLib_Browser/Logic Operations Changed/Relational Operator  Operator=<=  InputSameDT=on  LogicOutDataTypeMode=Specify via dialog  LogicDataType=PDT_Bool  OutDataTypeStr=PDT_Bool
  y : Outport
  wires:
  u/1 -> Relational Operator/1
  Constant/1 -> Relational Operator/2
  Relational Operator/1 -> y/1

== system PES_CZ_FAW/Math_and_Discrete/Compare To Zero ==
  u : Inport
  Constant : BaseOperationLib_Browser/Sources&Sinks/Constant  Value=0  OutMin=[]  OutMax=[]  OutDataType=fixdt(1, 16)  ConRadixGroup=Use specified scaling  OutScaling=2^0  OutDataTypeStr=Inherit: Inherit from 'Constant value'
  Relational Operator : BaseOperationLib_Browser/Logic Operations Changed/Relational Operator  Operator=<=  InputSameDT=on  LogicOutDataTypeMode=Specify via dialog  LogicDataType=PDT_Bool  OutDataTypeStr=PDT_Bool
  y : Outport
  wires:
  u/1 -> Relational Operator/1
  Constant/1 -> Relational Operator/2
  Relational Operator/1 -> y/1

== system PES_CZ_FAW/Math_and_Discrete/Detect Decrease ==
  U : Inport
  Relational Operator : RelationalOperator  Operator=<  LogicOutDataTypeMode=Specify via dialog  LogicDataType=PDT_Bool  OutDataTypeStr=PDT_Bool  InputSameDT=on
      mask Display: patch([0 1 1 1 .75], [1 1 0 .75 1], [0 1 0]);
  Unit Delay : UnitDelay  X0=vinit  SampleTime=-1
      mask Display: patch([0 1 1 1 .75], [1 1 0 .75 1], [0 1 0]);
  Y : Outport
  wires:
  U/1 -> Relational Operator/1, Unit Delay/1
  Unit Delay/1 -> Relational Operator/2
  Relational Operator/1 -> Y/1

== system PES_CZ_FAW/Math_and_Discrete/Range Check  ==
  in : Inport
  Constant : BaseOperationLib_Browser/Sources&Sinks/Constant  Value=Max  OutMin=[]  OutMax=[]  OutDataType=fixdt(1, 16)  ConRadixGroup=Use specified scaling  OutScaling=2^0  OutDataTypeStr=Inherit: Inherit from 'Constant value'
  Constant1 : BaseOperationLib_Browser/Sources&Sinks/Constant  Value=Min  OutMin=[]  OutMax=[]  OutDataType=fixdt(1, 16)  ConRadixGroup=Use specified scaling  OutScaling=2^0  OutDataTypeStr=Inherit: Inherit from 'Constant value'
  Logical Operator : BaseOperationLib_Browser/Logic Operations Changed/Logical Operator  Operator=AND  Inputs=2  AllPortsSameDT=on  OutDataTypeMode=Specify via dialog  LogicDataType=PDT_Bool  OutDataTypeStr=PDT_Bool
  Relational Operator1 : BaseOperationLib_Browser/Logic Operations Changed/Relational Operator  Operator=>=  InputSameDT=on  LogicOutDataTypeMode=Specify via dialog  LogicDataType=PDT_Bool  OutDataTypeStr=PDT_Bool
  Relational Operator2 : BaseOperationLib_Browser/Logic Operations Changed/Relational Operator  Operator=<=  InputSameDT=on  LogicOutDataTypeMode=Specify via dialog  LogicDataType=PDT_Bool  OutDataTypeStr=PDT_Bool
  out : Outport
  wires:
  Logical Operator/1 -> out/1
  Constant/1 -> Relational Operator2/2
  in/1 -> Relational Operator1/1, Relational Operator2/1
  Constant1/1 -> Relational Operator1/2
  Relational Operator2/1 -> Logical Operator/2
  Relational Operator1/1 -> Logical Operator/1

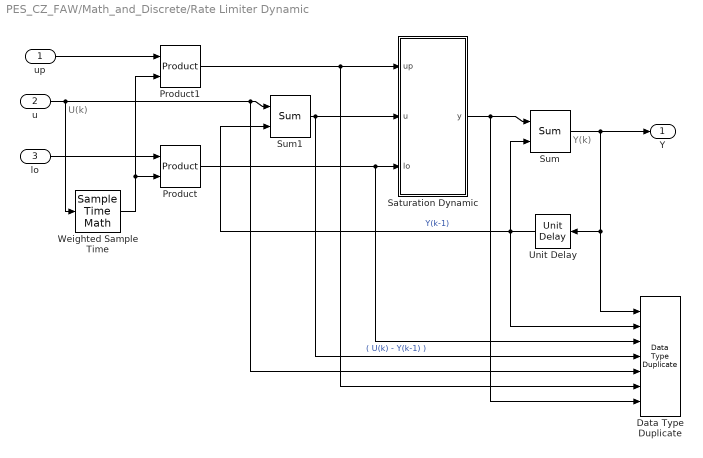
== system PES_CZ_FAW/Math_and_Discrete/Rate Limiter Dynamic ==
  note: Y(k)
  note: U(k)
  up : Inport  OutDataType=fixdt(1, 16)  OutScaling=2^0
  u : Inport  Port=2  OutDataType=fixdt(1, 16)  OutScaling=2^0
  lo : Inport  Port=3  OutDataType=fixdt(1, 16)  OutScaling=2^0
  Data Type Duplicate : DataTypeDuplicate  NumInputPorts=7
  Product : BaseOperationLib_Browser/Math Operations Changed/Product  Inputs=2  Multiplication=Element-wise(.*)  OutMin=[]  OutMax=[]  OutDataType=fixdt(1,16,0)  OutScaling=[]  OutDataTypeStr=Inherit: Inherit via back propagation  RndMeth=Zero  SaturateOnIntegerOverflow=on
  Product1 : BaseOperationLib_Browser/Math Operations Changed/Product  Inputs=2  Multiplication=Element-wise(.*)  OutMin=[]  OutMax=[]  OutDataType=fixdt(1,16,0)  OutScaling=[]  OutDataTypeStr=Inherit: Inherit via back propagation  RndMeth=Zero  SaturateOnIntegerOverflow=on
  Saturation Dynamic : Subsystem  mask(Saturation Dynamic){OutMin=[], OutMax=[], OutDataTypeStr=Inherit: Same as second input, OutputDataTypeScalingMode=Same as second input, OutDataType=fixdt(1, 16), OutScaling=2^-10, LockScale=off, RndMeth=Floor, DoSatur=off}
      mask prompts: OutMin "Output minimum:"; OutMax "Output maximum:"; OutDataTypeStr "Output data type:"; OutputDataTypeScalingMode "Output data type mode:"; OutDataType "Output data type (e.g. fixdt(1, 16), fixdt('single')):"; OutScaling "Output scaling (Slope, e.g. 2^-9 or [Slope Bias], e.g. [1.25 3]):"; LockScale "Lock output data type setting against changes by the fixed-point tools"; RndMeth "Integer rounding mode:"; DoSatur "Saturate on integer overflow"
      mask help: Bound the range of the second input by using the first input (upper limit) and the third input (lower limit).
      mask init:
      | blkH = gcbh;
      | blkName = getfullname(blkH);
      | 
      | switch_blks = {'Switch','Switch2'}; 
      | for i = 1:length(switch_blks)
      |   set_param([blkName,'/',switch_blks{i}], ...
      |       'RndMeth', RndMeth, ...
      | 	  'DoSatur', DoSatur);
      | end
      | 
      | propBlk = [blkName, '/Data Type Propagation'];
      | 
      | if strcmp(OutputDataTypeScalingMode, 'Same as second input')
      |     set_param(propBlk, 'PropDataTypeMode', 'Inherit via propagation rule', ...
      |                        'PropScalingMode',  'Inherit via propagation rule');
      | else
      |     scaling = OutScaling;
      |     switch OutputDataTypeScalingMode
      |       case 'double'
      |         dataType = 'fixdt(''double'')';
      |       case 'single'
      |         dataType = 'fixdt(''single'')';
      |       case 'int8'
      |         dataType = 'fixdt(1,8,0)';
      |       case 'uint8'
      |         dataType = 'fixdt(0,8,0)';
      |       case 'int16'
      |         dataType = 'fixdt(1,16,0)';
      |       case 'uint16'
      |         dataType = 'fixdt(0,16,0)';
      |       case 'int32'
      |         dataType = 'fixdt(1,32,0)';
      |       case 'uint32'
      |         dataType = 'fixdt(0,32,0)';
      |       case 'Specify via dialog'
      |         dataType = OutDataType;
      |     end
      |     
      |     set_param(propBlk, 'PropDataTypeMode', 'Specify via dialog', ...
      |                        'PropScalingMode',  'Specify via dialog', ...
      |                        'PropDataType',     dataType, ...
      |                        'PropScaling',      scaling);
      | end
      mask StyleString: min,max,unidt({m=3|4|5||6|1|2|}{i=Inherit: Same as second input}{b=double|single|int8|uint8|int16|uint16|int32|uint32}{s=UDTBinaryPointMode|UDTSlopeBiasMode}{g=UDTSignedSign|UDTUnsignedSign}),popup(double|single|int8|uint8|int16|uint16|int32|uint32|Specify via dialog|Same as second input),edit,edit,checkbox,popup(Ceiling|Convergent|Floor|Nearest|Round|Simplest|Zero),checkbox
      mask CallbackString: ||fixptdialog(gcbh)|fixptdialog(gcbh)|fixptdialog(gcbh)||||
      mask TabNameString: Signal Attributes,Signal Attributes,Signal Attributes,Signal Attributes,Signal Attributes,Signal Attributes,Signal Attributes,Signal Attributes,Signal Attributes
      mask Display: plot([0.15 0.85],[.5 .5],[.5 .5],[0.05 0.95],0.15+0.7*[0 .25 .75 1],0.05+0.9*[.25 .25 .75 .75]);
  Sum : BaseOperationLib_Browser/Math Operations Changed/Sum  Inputs=++  InputSameDT=on  OutMin=[]  OutMax=[]  OutDataType=fixdt(1, 16)  OutScaling=2^0  SaturateOnIntegerOverflow=on
  Sum1 : BaseOperationLib_Browser/Math Operations Changed/Sum  Inputs=+-  InputSameDT=on  OutMin=[]  OutMax=[]  OutDataType=fixdt(1, 16)  OutScaling=2^0  SaturateOnIntegerOverflow=on
  Unit Delay : BaseOperationLib_Browser/Discrete Unchanged /Unit Delay  X0=0  SampleTime=-1
  Weighted Sample Time : SampleTimeMath  TsampMathOp=Ts Only  weightValue=1
  Y : Outport
  wires:
  Sum1/1 -> Saturation Dynamic/2(u), Data Type Duplicate/4  "( U(k) - Y(k-1) )"
  u/1 -> Weighted Sample Time/1, Sum1/1, Data Type Duplicate/5
  Product/1 -> Saturation Dynamic/3(lo), Data Type Duplicate/3
  Saturation Dynamic/1(y) -> Sum/1, Data Type Duplicate/7
  Unit Delay/1 -> Sum/2, Sum1/2, Data Type Duplicate/2  "Y(k-1)"
  Sum/1 -> Y/1, Unit Delay/1, Data Type Duplicate/1
  up/1 -> Product1/1
  Product1/1 -> Saturation Dynamic/1(up), Data Type Duplicate/6
  lo/1 -> Product/1
  Weighted Sample Time/1 -> Product1/2, Product/2

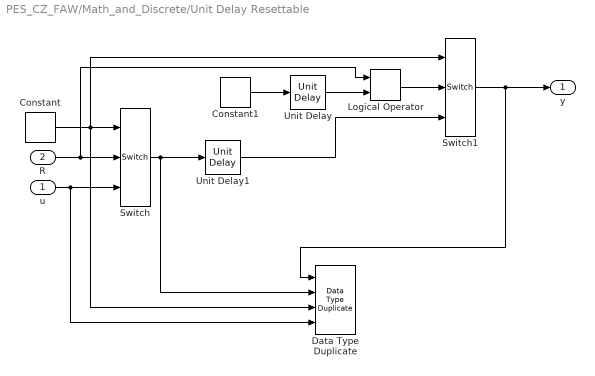
== system PES_CZ_FAW/Math_and_Discrete/Unit Delay Resettable ==
  u : Inport
  R : Inport  Port=2
  Constant : BaseOperationLib_Browser/Sources&Sinks/Constant  Value=vinit  OutMin=[]  OutMax=[]  OutDataType=fixdt(1, 16)  ConRadixGroup=Use specified scaling  OutScaling=2^0  OutDataTypeStr=Inherit: Inherit via back propagation
  Constant1 : BaseOperationLib_Browser/Sources&Sinks/Constant  Value=0  OutMin=[]  OutMax=[]  OutDataType=fixdt(1, 16)  ConRadixGroup=Use specified scaling  OutScaling=2^0  OutDataTypeStr=Inherit: Inherit via back propagation
  Data Type Duplicate : DataTypeDuplicate  NumInputPorts=4
  Logical Operator : BaseOperationLib_Browser/Logic Operations Changed/Logical Operator  Operator=OR  Inputs=2  AllPortsSameDT=on  OutDataTypeMode=Specify via dialog  LogicDataType=PDT_Bool  OutDataTypeStr=PDT_Bool
  Switch : BaseOperationLib_Browser/Signal Routing Changed/Switch  Criteria=u2 ~= 0  Threshold=1  InputSameDT=on  OutMin=[]  OutMax=[]  OutDataType=fixdt(1,16,0)  OutScaling=[]  SaturateOnIntegerOverflow=on
  Switch1 : BaseOperationLib_Browser/Signal Routing Changed/Switch  Criteria=u2 ~= 0  Threshold=1  InputSameDT=on  OutMin=[]  OutMax=[]  OutDataType=fixdt(1,16,0)  OutScaling=[]  SaturateOnIntegerOverflow=on
  Unit Delay : BaseOperationLib_Browser/Discrete Unchanged /Unit Delay  X0=1  SampleTime=tsamp
  Unit Delay1 : BaseOperationLib_Browser/Discrete Unchanged /Unit Delay  X0=vinit  SampleTime=tsamp
  y : Outport
  wires:
  Switch1/1 -> Data Type Duplicate/1, y/1
  Unit Delay1/1 -> Switch1/3
  Switch/1 -> Data Type Duplicate/2, Unit Delay1/1
  Logical Operator/1 -> Switch1/2
  Unit Delay/1 -> Logical Operator/2
  Constant1/1 -> Unit Delay/1
  Constant/1 -> Data Type Duplicate/3, Switch1/1, Switch/1
  u/1 -> Data Type Duplicate/4, Switch/3
  R/1 -> Logical Operator/1, Switch/2
